simulink model "Bilateral_teleoperation_compensation"  (R2017a)
settings: Solver=FixedStepAuto  StartTime=0.0  StopTime=5  FixedStep=0.005  RelTol=1e-3  EnableMultiTasking=on
libraries: arduinolib x7, simulink x4
settings Model: SimulationMode=external  ExtModeTrigDuration=2  Creator=juanma  LastModifiedBy=juanma
settings OptimizationCC: PassReuseOutputArgsAs=Individual arguments  MaxStackSize=64
settings DebuggingCC: IntegerOverflowMsg=none  ParameterOverflowMsg=none  ParameterTunabilityLossMsg=error  IntegerSaturationMsg=none
settings HardwareCC: ProdBitPerInt=16  ProdBitPerPointer=16  ProdBitPerSizeT=16  ProdBitPerPtrDiffT=16  ProdLargestAtomicFloat=None  ProdWordSize=8  ProdHWDeviceType=Atmel->AVR
settings SFSimCC: MATLABDynamicMemAlloc=off
settings RTWCC: SystemTargetFile=ert.tlc  HardwareBoard=Arduino Mega 2560  TLCOptions=-aInlineSetEventsForThisBaseRateFcn=TLC_FALSE -aSuppressMultiTaskScheduler=TLC_FALSE -aRateBasedStepFcn=1  TemplateMakefile=ert_default_tmf  Description=Embedded Coder  GenerateReport=on  Toolchain=Arduino AVR  BuildConfiguration=Faster Runs  IncludeHyperlinkInReport=on  LaunchReport=on  GenerateTraceInfo=on  GenerateTraceReport=on  GenerateTraceReportSl=on  GenerateTraceReportSf=on  GenerateTraceReportEml=on
settings CodeAppCC: ForceParamTrailComments=on  IgnoreCustomStorageClasses=off  OperatorAnnotations=on  SimulinkDataObjDesc=on  SFDataObjDesc=on  MATLABFcnDesc=on  InsertBlockDesc=on  MATLABSourceComments=on
settings ERTTargetCC: SupportContinuousTime=on  SupportVariableSizeSignals=on

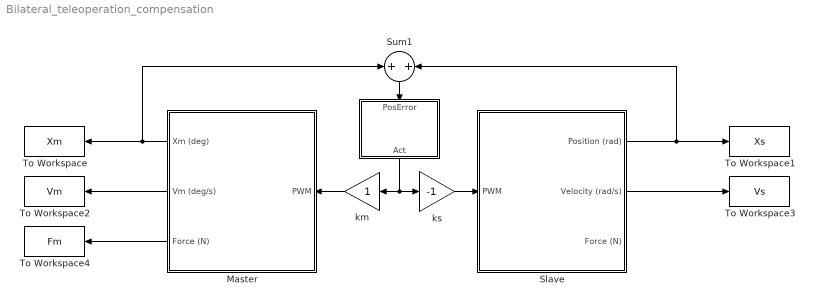
== system Bilateral_teleoperation_compensation ==
  " " : Subsystem
      mask Display: disp('G(s)')
  Master : Subsystem
      mask Display:
      | pic=imread('haptic2017_render.png');
      | image(pic);
      | % color('blue');
      | % text(10, 10, 'HapticMega');
      | color('black');
      | port_label('Input', 1, 'PWM');
      | port_label('Output', 1, 'Position (deg)');
      | port_label('Output', 2, 'Velocity (deg/s)');
      | port_label('Output', 3, 'Force (N)');
  Slave : Subsystem
      mask Display:
      | pic=imread('haptic2017_render.png');
      | image(pic);
      | % color('blue');
      | % text(10, 10, 'HapticMega');
      | color('black');
      | port_label('Input', 1, 'PWM');
      | port_label('Output', 1, 'Position (deg)');
      | port_label('Output', 2, 'Velocity (deg/s)');
      | port_label('Output', 3, 'Force (N)');
  Sum1 : Sum  Inputs=+|+
  To Workspace : ToWorkspace  VariableName=Xm  SaveFormat=Structure With Time  SampleTime=-1
  To Workspace1 : ToWorkspace  VariableName=Xs  SaveFormat=Structure With Time  SampleTime=-1
  To Workspace2 : ToWorkspace  VariableName=Vm  SaveFormat=Structure With Time  SampleTime=-1
  To Workspace3 : ToWorkspace  VariableName=Vs  SaveFormat=Structure With Time  SampleTime=-1
  To Workspace4 : ToWorkspace  VariableName=Fm  SaveFormat=Structure With Time  SampleTime=-1
  km : Gain  OutDataTypeStr=int16
  ks : Gain  Gain=-1  OutDataTypeStr=int16
  wires:
  Master/1(Xm (deg)) -> To Workspace/1, Sum1/1
  Slave/1(Position (rad)) -> To Workspace1/1, Sum1/2
  " "/1(Act) -> ks/1, km/1
  ks/1 -> Slave/1(PWM)
  km/1 -> Master/1(PWM)
  Sum1/1 -> " "/1(PosError)
  Master/3(Force (N)) -> To Workspace4/1
  Master/2(Vm (deg/s)) -> To Workspace2/1
  Slave/2(Velocity (rad/s)) -> To Workspace3/1

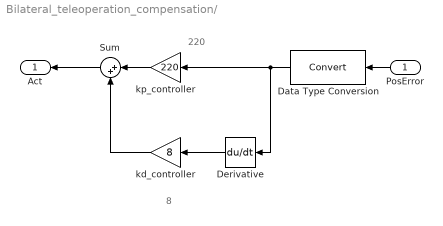
== system Bilateral_teleoperation_compensation/  ==
  note: 220
  note: 8
  PosError : Inport
  Data Type Conversion : DataTypeConversion
  Derivative : Derivative
  Sum : Sum  Inputs=|++
  kd_controller : Gain  Gain=8
  kp_controller : Gain  Gain=220
  Act : Outport
  wires:
  PosError/1 -> Data Type Conversion/1
  kp_controller/1 -> Sum/1
  Sum/1 -> Act/1
  Data Type Conversion/1 -> kp_controller/1, Derivative/1
  Derivative/1 -> kd_controller/1
  kd_controller/1 -> Sum/2

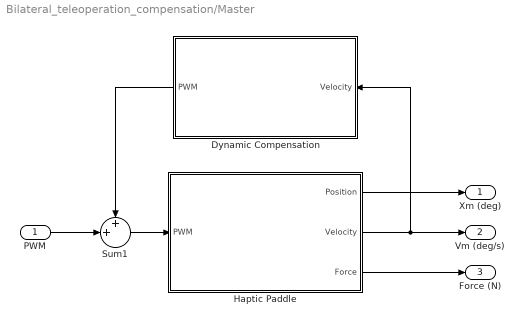
== system Bilateral_teleoperation_compensation/Master ==
  PWM : Inport  OutDataTypeStr=int16
  Dynamic Compensation : Subsystem
  Haptic Paddle : Subsystem
  Sum1 : Sum  Inputs=++|
  Xm (deg) : Outport
  Vm (deg/s) : Outport  Port=2
  Force (N) : Outport  Port=3
  wires:
  Haptic Paddle/1(Position) -> Xm (deg)/1
  Haptic Paddle/2(Velocity) -> Vm (deg/s)/1, Dynamic Compensation/1(Velocity)
  Haptic Paddle/3(Force) -> Force (N)/1
  Sum1/1 -> Haptic Paddle/1(PWM)
  Dynamic Compensation/1(PWM) -> Sum1/1
  PWM/1 -> Sum1/2

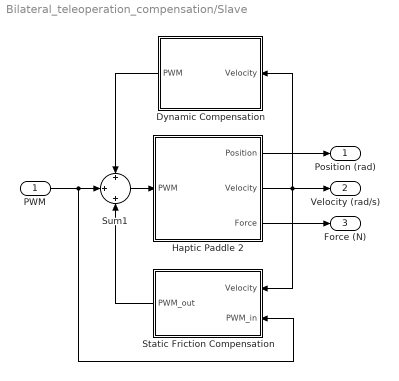
== system Bilateral_teleoperation_compensation/Slave ==
  PWM : Inport
  Dynamic Compensation : Subsystem
  "Haptic Paddle 2 " : Subsystem
  Static Friction Compensation : Subsystem
  Sum1 : Sum  Inputs=+|+|+
  Position (rad) : Outport
  Velocity (rad/s) : Outport  Port=2
  Force (N) : Outport  Port=3
  wires:
  "Haptic Paddle 2 "/1(Position) -> Position (rad)/1
  "Haptic Paddle 2 "/3(Force) -> Force (N)/1
  "Haptic Paddle 2 "/2(Velocity) -> Dynamic Compensation/1(Velocity), Velocity (rad/s)/1, Static Friction Compensation/1(Velocity)
  Dynamic Compensation/1("PWM ") -> Sum1/1
  PWM/1 -> Static Friction Compensation/2(PWM_in), Sum1/2
  Sum1/1 -> "Haptic Paddle 2 "/1("PWM ")
  Static Friction Compensation/1(PWM_out) -> Sum1/3

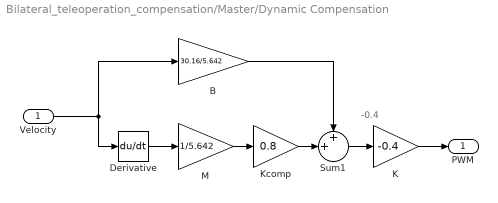
== system Bilateral_teleoperation_compensation/Master/Dynamic Compensation ==
  note: -0.4
  Velocity : Inport
  B : Gain  Gain=30.16/5.642  OutDataTypeStr=double
  Derivative : Derivative
  K : Gain  Gain=-0.4  OutDataTypeStr=int16
  Kcomp : Gain  Gain=0.8  OutDataTypeStr=int16
  M : Gain  Gain=1/5.642  OutDataTypeStr=double
  Sum1 : Sum  Inputs=++|
  PWM : Outport
  wires:
  Sum1/1 -> K/1
  B/1 -> Sum1/1
  Derivative/1 -> M/1
  Velocity/1 -> Derivative/1, B/1
  M/1 -> Kcomp/1
  K/1 -> PWM/1
  Kcomp/1 -> Sum1/2

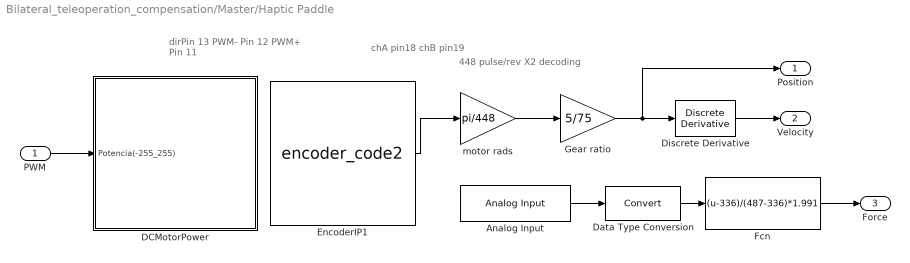
== system Bilateral_teleoperation_compensation/Master/Haptic Paddle ==
  note: dirPin 13
      | PWM- Pin 12
      | PWM+ Pin 11
  note: chA pin18
      | chB pin19
  note: 448 pulse/rev
      | X2 decoding
  PWM : Inport
  Analog Input : arduinolib/Analog Input  pinNumber=8  sampleTime=-1  blockPlatform=arduino
  DCMotorPower : Subsystem
      settings: RTWFcnNameOpts=Use subsystem name  RTWFileNameOpts=Use function name
      mask Display:
      | pic=imread('L298.jpg');
      | image(pic,[0.28 0.18 0.45 0.65]);
      | 
      | color('blue');
      | text(0.1, 0.87, 'Puente H', 'horizontalAlignment', 'left');
      | color('black');
      | port_label('Input', 1, 'PWM');
  Data Type Conversion : DataTypeConversion
  Discrete Derivative : simulink/Discrete/Discrete Derivative  gainval=1  ICPrevScaledInput=0.0  InputProcessing=Inherited  OutMin=[]  OutMax=[]  OutDataTypeStr=double  OutputDataTypeScalingMode=double  OutDataType=fixdt(1, 16)  OutScaling=2^-10  DoSatur=off
  EncoderIP1 : S-Function  InitFcn=try, set_param(gcb,'FunctionName','encoder_code2'), end  FunctionName=encoder_code2  Parameters=uint8(1),uint8(18),uint8(19)  SFunctionModules=encoder_code2_wrapper  SFunctionDeploymentMode=off  EnableBusSupport=off  mask(S-Function Builder){}
      mask init:
      | val = [[.9  0.75 0.75 1 1 .9 .9 1]',[1 1 0.75 0.75 .9 .9 1 .9]'];try , sys = get_param(gcb,'SfunBuilderFcnName');if isempty(sys), sys = get_param(gcb,'FunctionName'); end,catch, sys = get_param(gcb,'FunctionName'); end
      settings: CopyFcn=set_param(gcbh,'LinkStatus','none')  PreSaveFcn=try, set_param(gcb,'FunctionName','encoder_code2'), end  OpenFcn=sfunctionwizard(gcbh)
      mask Display: plot(val(:,1),val(:,2)),disp(sys), port_label('output',1,'pos')
  Fcn : Fcn  Expr=(u-336)/(487-336)*1.991
  "Gear ratio " : Gain  Gain=5/75
  motor rads : Gain  Gain=pi/448
  Position : Outport
  Velocity : Outport  Port=2
  Force : Outport  Port=3
  wires:
  Discrete Derivative/1 -> Velocity/1
  motor rads/1 -> "Gear ratio "/1
  PWM/1 -> DCMotorPower/1("Potencia(-255_255) ")
  EncoderIP1/1 -> motor rads/1
  "Gear ratio "/1 -> Position/1, Discrete Derivative/1
  Data Type Conversion/1 -> Fcn/1
  Analog Input/1 -> Data Type Conversion/1
  Fcn/1 -> Force/1

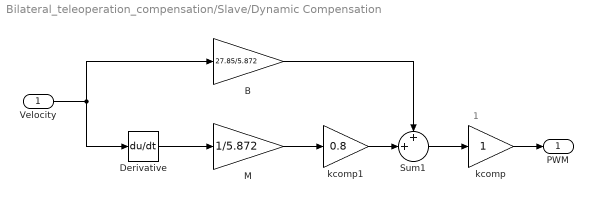
== system Bilateral_teleoperation_compensation/Slave/Dynamic Compensation ==
  note: 1
  Velocity : Inport
  B : Gain  Gain=27.85/5.872  OutDataTypeStr=double
  Derivative : Derivative
  M : Gain  Gain=1/5.872  OutDataTypeStr=double
  Sum1 : Sum  Inputs=++|
  kcomp : Gain  OutDataTypeStr=int16
  kcomp1 : Gain  Gain=0.8  OutDataTypeStr=int16
  "PWM " : Outport
  wires:
  M/1 -> kcomp1/1
  B/1 -> Sum1/1
  Velocity/1 -> B/1, Derivative/1
  Derivative/1 -> M/1
  Sum1/1 -> kcomp/1
  kcomp/1 -> "PWM "/1
  kcomp1/1 -> Sum1/2

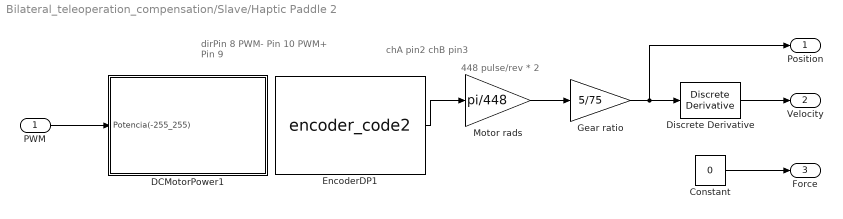
== system Bilateral_teleoperation_compensation/Slave/Haptic Paddle 2  ==
  note: dirPin 8
      | PWM- Pin 10
      | PWM+ Pin 9
  note: chA pin2
      | chB pin3
  note: 448 pulse/rev * 2
  "PWM " : Inport
  Constant : Constant  Value=0
  DCMotorPower1 : Subsystem
      settings: RTWFcnNameOpts=Use subsystem name  RTWFileNameOpts=Use function name
      mask Display:
      | pic=imread('L298.jpg');
      | image(pic,[0.28 0.18 0.45 0.65]);
      | 
      | color('blue');
      | text(0.1, 0.87, 'Puente H', 'horizontalAlignment', 'left');
      | color('black');
      | port_label('Input', 1, 'PWM');
  Discrete Derivative : simulink/Discrete/Discrete Derivative  gainval=1  ICPrevScaledInput=0.0  InputProcessing=Inherited  OutMin=[]  OutMax=[]  OutDataTypeStr=double  OutputDataTypeScalingMode=double  OutDataType=fixdt(1, 16)  OutScaling=2^-10  DoSatur=off
  EncoderDP1 : S-Function  InitFcn=try, set_param(gcb,'FunctionName','encoder_code2'), end  FunctionName=encoder_code2  Parameters=uint8(0),uint8(2),uint8(3)  SFunctionModules=encoder_code2_wrapper  SFunctionDeploymentMode=off  EnableBusSupport=off  mask(S-Function Builder){}
      mask init: same as Bilateral_teleoperation_compensation/Master/Haptic Paddle/EncoderIP1
      settings: CopyFcn=set_param(gcbh,'LinkStatus','none')  PreSaveFcn=try, set_param(gcb,'FunctionName','encoder_code2'), end  OpenFcn=sfunctionwizard(gcbh)
      mask Display: plot(val(:,1),val(:,2)),disp(sys), port_label('output',1,'pos')
  "Gear ratio " : Gain  Gain=5/75
  Motor rads : Gain  Gain=pi/448
  Position : Outport
  Velocity : Outport  Port=2
  Force : Outport  Port=3
  wires:
  Constant/1 -> Force/1
  Motor rads/1 -> "Gear ratio "/1
  EncoderDP1/1 -> Motor rads/1
  Discrete Derivative/1 -> Velocity/1
  "PWM "/1 -> DCMotorPower1/1("Potencia(-255_255) ")
  "Gear ratio "/1 -> Position/1, Discrete Derivative/1

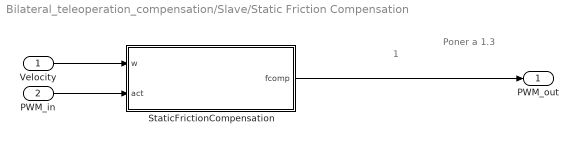
== system Bilateral_teleoperation_compensation/Slave/Static Friction Compensation ==
  note: 1
  note: Poner a 1.3
  Velocity : Inport
  PWM_in : Inport  Port=2
  StaticFrictionCompensation : MATLAB Function  TreatAsAtomicUnit=on
  PWM_out : Outport
  wires:
  Velocity/1 -> StaticFrictionCompensation/1(w)
  PWM_in/1 -> StaticFrictionCompensation/2(act)
  StaticFrictionCompensation/1(fcomp) -> PWM_out/1

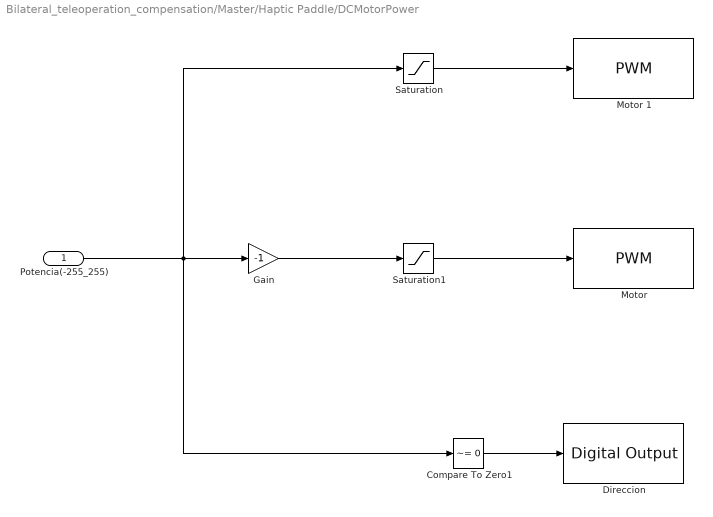
== system Bilateral_teleoperation_compensation/Master/Haptic Paddle/DCMotorPower ==
  "Potencia(-255_255) " : Inport  OutDataTypeStr=int16
  Compare To Zero1 : simulink/Logic and Bit Operations/Compare To Zero  relop=~=  OutDataTypeStr=boolean
  Direccion : arduinolib/Digital Output  pinNumber=13  blockPlatform=arduino
  Gain : Gain  Gain=-1
  Motor : arduinolib/PWM  pinNumber=11  blockPlatform=arduino
  Motor 1 : arduinolib/PWM  pinNumber=12  blockPlatform=arduino
  Saturation : Saturate  UpperLimit=255  LowerLimit=0
  Saturation1 : Saturate  UpperLimit=255  LowerLimit=0
  wires:
  Saturation/1 -> Motor 1/1
  Compare To Zero1/1 -> Direccion/1
  Saturation1/1 -> Motor/1
  Gain/1 -> Saturation1/1
  "Potencia(-255_255) "/1 -> Saturation/1, Compare To Zero1/1, Gain/1

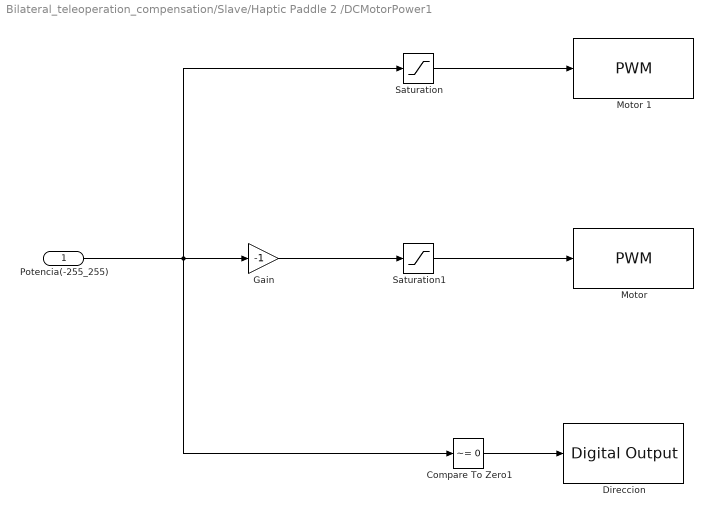
== system Bilateral_teleoperation_compensation/Slave/Haptic Paddle 2 /DCMotorPower1 ==
  "Potencia(-255_255) " : Inport  OutDataTypeStr=int16
  Compare To Zero1 : simulink/Logic and Bit Operations/Compare To Zero  relop=~=  OutDataTypeStr=boolean
  Direccion : arduinolib/Digital Output  pinNumber=8  blockPlatform=arduino
  Gain : Gain  Gain=-1
  Motor : arduinolib/PWM  pinNumber=10  blockPlatform=arduino
  Motor 1 : arduinolib/PWM  pinNumber=9  blockPlatform=arduino
  Saturation : Saturate  UpperLimit=255  LowerLimit=0
  Saturation1 : Saturate  UpperLimit=255  LowerLimit=0
  wires:
  Saturation/1 -> Motor 1/1
  Compare To Zero1/1 -> Direccion/1
  Saturation1/1 -> Motor/1
  Gain/1 -> Saturation1/1
  "Potencia(-255_255) "/1 -> Saturation/1, Compare To Zero1/1, Gain/1

== matlab function Bilateral_teleoperation_compensation/Slave/Static Friction Compensation/StaticFrictionCompensation ==
  data: w input; fcomp output; act input
function fcomp = StaticCompensation(w, act)
    %Static Friction Estimation
    fs = 20;
    %We've to consider the velocity's noise
    %If exist an error and the velocity is ~0, but the actuation signal is
    %<60, which could mean there is a contact on the other haptic
    if (abs(act)>0)&&((abs(w)<=0.1))&&(abs(act)<=fs) 
        fcomp = fs*sign(act);
    else
        fcomp = int16(0);
    end
end
